simulink model "Copy_of_Controller"  (R2023a)
settings: Solver=FixedStepDiscrete  StartTime=0.0  StopTime=inf  FixedStep=0.001  RelTol=1e-3  EnableMultiTasking=on
undefined symbols (not defined in the file): den_d, num_d
libraries: quarc_library x4
settings Model: SimulationMode=external  ExtModeTrigType=signal  ExtModeTrigDuration=60000  ExtModeTrigDirection=either  ExtModeTrigLevel=0.500000  Creator=colegiusto  LastModifiedBy=colegiusto
settings SolverCC: PositivePriorityOrder=on
settings RTWCC: Description=QUARC Win64 Target Using Toolchain  SystemTargetFile=quarc_win64.tlc  Toolchain=QUARC win64 | nmake (64-bit Windows)  BuildConfiguration=Faster Runs
settings STFCustomTargetCC: TargetLangStandard=C89/C90 (ANSI)  SystemTargetFile=quarc_win64.tlc
settings GRTTargetCC: TargetLangStandard=C89/C90 (ANSI)  ParMdlRefBuildCompliant=off  CompOptLevelCompliant=off  CombineOutputUpdateFcns=off  MatFileLogging=off  CPPClassGenCompliant=off  GRTInterface=on  ExtMode=on  ExtModeMexFile=quarc_comm

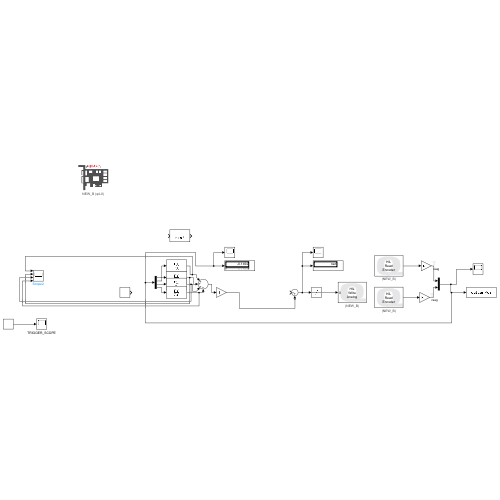
[thumbnail: Simulink's stored preview of the top-level diagram]
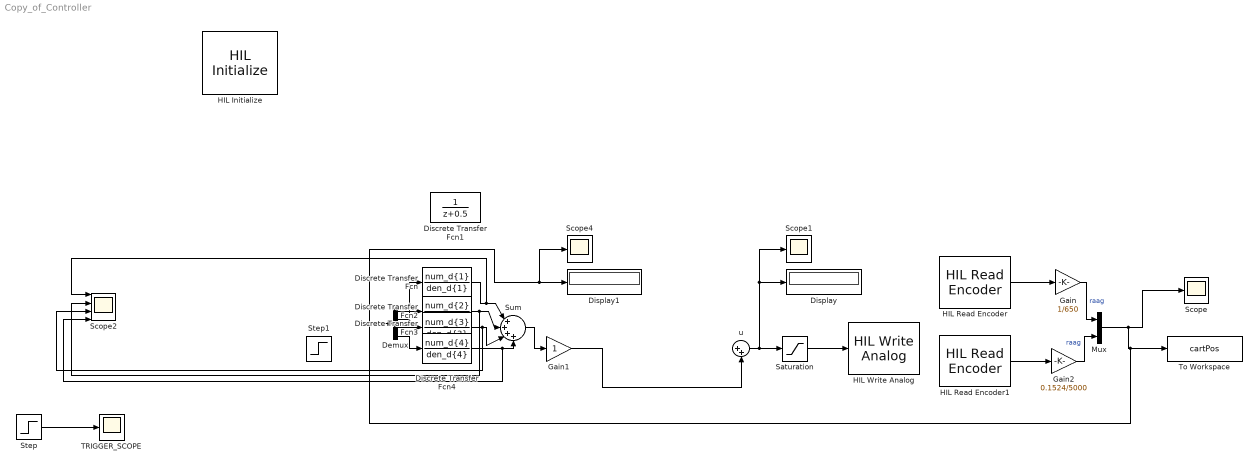
== system Copy_of_Controller ==
  Demux : Demux
  Discrete Transfer Fcn : DiscreteTransferFcn  Numerator=num_d{1}  Denominator=den_d{1}  SampleTime=0.001
  Discrete Transfer Fcn1 : DiscreteTransferFcn
  Discrete Transfer Fcn2 : DiscreteTransferFcn  Numerator=num_d{2}  Denominator=den_d{2}  SampleTime=0.001
  Discrete Transfer Fcn3 : DiscreteTransferFcn  Numerator=num_d{3}  Denominator=den_d{3}  SampleTime=0.001
  Discrete Transfer Fcn4 : DiscreteTransferFcn  Numerator=num_d{4}  Denominator=den_d{4}  SampleTime=0.001
  Display : Display
  Display1 : Display
  Gain : Gain  Gain=1/650
  Gain1 : Gain
  Gain2 : Gain  Gain=0.1524/5000
  HIL Initialize : quarc_library/Data Acquisition/Generic/Configuration/HIL Initialize  object_name=NEW_B  board_type=q4  board_number=0  board_options=""  exclusive=off  active=on  hardware_clocks=[0:1]  clock_modes=[0 0]  initial_clock_frequencies=[]  set_clock_params_at_start=on  set_clock_params_at_switch_in=off  set_clock_frequencies_at_start=off  set_clock_frequencies_at_switch_in=off  analog_input_channels=[0:3]  analog_input_configurations=[]  analog_input_maximums=10  analog_input_minimums=-10  set_analog_input_params_at_start=off  set_analog_input_params_at_switch_in=off  analog_output_channels=[0:3]  analog_output_maximums=[10]  analog_output_minimums=[-10]  initial_analog_outputs=[0]  final_analog_outputs=[0]  watchdog_analog_outputs=0  set_analog_output_params_at_start=on  set_analog_output_params_at_switch_in=off  set_analog_outputs_at_start=on  set_analog_outputs_at_switch_in=off  set_analog_outputs_at_terminate=on  set_analog_outputs_at_switch_out=off  set_analog_outputs_on_watchdog=off  digital_input_channels=[]  digital_output_channels=[]  digital_output_configuration=[]  initial_digital_outputs=[1]  final_digital_outputs=[1]  watchdog_digital_outputs=[2]  set_digital_output_params_at_start=off  set_digital_output_params_at_switch_in=off  set_digital_outputs_at_start=on  set_digital_outputs_at_switch_in=off  set_digital_outputs_at_terminate=on  set_digital_outputs_at_switch_out=off  set_digital_outputs_on_watchdog=off  encoder_channels=[0:3]  quadrature=[4]  encoder_filter_frequency=(1/60e-9)/1  initial_encoder_counts=[0]  set_encoder_params_at_start=on  set_encoder_params_at_switch_in=off  set_encoder_counts_at_start=on  set_encoder_counts_at_switch_in=off  pwm_channels=[]  pwm_modes=[0]  pwm_frequency=(1/60e-9)/1024  pwm_configuration=[]  pwm_alignment=[]  pwm_polarity=[]  pwm_leading_deadband=[]  pwm_trailing_deadband=[]  initial_pwm_outputs=[0]  final_pwm_outputs=[0]  watchdog_pwm_outputs=[]  set_pwm_params_at_start=on  set_pwm_params_at_switch_in=off  set_pwm_outputs_at_start=on  set_pwm_outputs_at_switch_in=off  set_pwm_outputs_at_terminate=on  set_pwm_outputs_at_switch_out=off  set_pwm_outputs_on_watchdog=off  other_output_channels=[]  initial_other_outputs=[]  final_other_outputs=[]  watchdog_other_outputs=[]  set_other_outputs_at_start=off  set_other_outputs_at_switch_in=off  set_other_outputs_at_terminate=off  set_other_outputs_at_switch_out=off  set_other_outputs_on_watchdog=off
  HIL Read Encoder : quarc_library/Data Acquisition/Generic/Immediate I//O/HIL Read Encoder  object_name=NEW_B  channels=[1, 3]  sample_time=0.001  active=on  vector_output=on  data_type_mode=Inherit via back propagation  data_type=double
  HIL Read Encoder1 : quarc_library/Data Acquisition/Generic/Immediate I//O/HIL Read Encoder  object_name=NEW_B  channels=[0,2]  sample_time=0.001  active=on  vector_output=on  data_type_mode=Inherit via back propagation  data_type=double
  HIL Write Analog : quarc_library/Data Acquisition/Generic/Immediate I//O/HIL Write Analog  object_name=NEW_B  channels=0  sample_time=0.001  active=off  vector_input=off
  Mux : Mux  Inputs=2
  Saturation : Saturate  UpperLimit=5  LowerLimit=-5
  Scope : Scope
  Scope1 : Scope
  Scope2 : Scope  NumInputPorts=4
  Scope4 : Scope
  Step : Step  Time=0.001  SampleTime=0
  Step1 : Step  After=0.3  SampleTime=0
  Sum : Sum  Inputs=|++++
  TRIGGER_SCOPE : Scope
  To Workspace : ToWorkspace  VariableName=cartPos  SaveFormat=Structure With Time  SampleTime=-1
  u : Sum  Inputs=|++
  wires:
  HIL Read Encoder/1 -> Gain/1
  Step/1 -> TRIGGER_SCOPE/1
  Gain/1 -> Mux/1  "raag"
  Mux/1 -> Demux/1, Scope4/1, Display1/1, To Workspace/1, Scope/1
  Saturation/1 -> HIL Write Analog/1
  u/1 -> Saturation/1, Scope1/1, Display/1
  Gain1/1 -> u/2
  HIL Read Encoder1/1 -> Gain2/1
  Gain2/1 -> Mux/2  "raag"
  Demux/1 -> Discrete Transfer Fcn/1
  Demux/2 -> Discrete Transfer Fcn2/1
  Demux/3 -> Discrete Transfer Fcn3/1
  Demux/4 -> Discrete Transfer Fcn4/1
  Sum/1 -> Gain1/1
  Discrete Transfer Fcn4/1 -> Scope2/4, Sum/4
  Discrete Transfer Fcn3/1 -> Scope2/3, Sum/3
  Discrete Transfer Fcn2/1 -> Sum/2, Scope2/2
  Discrete Transfer Fcn/1 -> Scope2/1, Sum/1
